simulink model "DoubleTankSim2023a"  (R2023a)
settings: Solver=ode5  StartTime=0.0  StopTime=250  RelTol=1e-3  EnableMultiTasking=on
values from neighbouring files (symbols this model uses):
  a1 = 0.145    [LeakSim.mat]    (also in disturbance.mat; main.m; mainLeak.m; out.mat)
  a2 = 0.145    [LeakSim.mat]    (also in disturbance.mat; main.m = 0.155; mainLeak.m; out.mat = 0.155)
  A_a = 33    [LeakSim.mat]    (also in disturbance.mat; main.m = 35; mainLeak.m; out.mat = 35)
  Ad = [0.997096423391  0  -0.448552524425; 0.00289935714461  0.997096423391  -0.000651834498432; 0  0  1]    [LeakSim.mat]    (also in disturbance.mat; out.mat = [0.998598500105  0; 0.00140036726045  0.998384495353]; out12.mat = [0.998598500105  0; 0.00140036726045  0.998384495353]; outLeak.mat = [0.998598500105  0; 0.00140036726045  0.998384495353])
  Bd = [0.0151295076986 2.19861321144e-05 0]    [LeakSim.mat]    (also in disturbance.mat; out.mat = [0.0107067759242 7.50574399214e-06]; out12.mat = [0.0107067759242 7.50574399214e-06]; outLeak.mat = [0.0107067759242 7.50574399214e-06])
  Cd = [0 1 0]    [LeakSim.mat]    (also in disturbance.mat; out.mat = [0 1]; out12.mat = [0 1]; outLeak.mat = [0 1])
  fh = [3 4 5 6 7 8 9 10 11 12 13 14 ... (13 elements, 1x13)]    [LeakSim.mat]    (also in disturbance.mat; main.m = [3 4 5 6 7 8 9 10 11 12 13 14 15]; mainLeak.m = [3 4 5 6 7 8 9 10 11 12 13 14 15]; out.mat)
  fq = [17.75 21.65 23.76 27.55 30.01 31.98 33.88 38.18 46.28 49.88]    [LeakSim.mat]    (also in disturbance.mat; main.m; mainLeak.m; out.mat)
  fu = [0.5 1 1.5 2 2.5 3 3.5 5 8 10]    [LeakSim.mat]    (also in disturbance.mat; main.m; mainLeak.m; out.mat)
  fv = [0.909 1.685 2.475 3.255 4.055 4.804 5.573 6.332 7.121 7.847 8.617 9.405 ... (13 elements, 1x13)]    [LeakSim.mat]    (also in disturbance.mat; main.m = [0.909 1.685 2.475 3.255 4.055 4.804 5.573 6.332 7.121 7.847; mainLeak.m = [0.909 1.685 2.475 3.255 4.055 4.804 5.573 6.332 7.121 7.847; out.mat)
  h0 = 3.2    [LeakSim.mat]    (also in disturbance.mat; main.m; mainLeak.m; out.mat)
  N = [1  0  0; 0  1  0; 0  0  1]    [LeakSim.mat]    (also in disturbance.mat; main.m = eye(2); mainLeak.m = eye(3); out.mat = [1  0; 0  1])
  P0 = [0  0  0; 0  0  0; 0  0  0]    [LeakSim.mat]    (also in disturbance.mat; main.m = zeros(2); mainLeak.m = zeros(3); out.mat = [0  0; 0  0])
  Q = [0.01  0  0; 0  0.01  0; 0  0  0.0001]    [LeakSim.mat]    (also in disturbance.mat; main.m = 0.1*eye(2); mainLeak.m = 0.01*eye(3,3); out.mat = [0.1  0; 0  0.1])
  R = 1e-06    [LeakSim.mat]    (also in disturbance.mat; main.m = Np*eye(2); mainLeak.m; out.mat = [0.0001  0; 0  0.0001])
  Ts = 0.1    [LeakSim.mat]    (also in disturbance.mat; main.m = 0.05; mainLeak.m; out.mat = 0.05)
  x0 = [-8 -8 0]    [LeakSim.mat]    (also in disturbance.mat; main.m = [0 0]'; mainLeak.m = [-8 -8 0]'; out.mat = [0 0])
undefined symbols (not defined in the file or in its folder): Continuous, Time
libraries: simulink x3, ctrlSharedLib x1
Description:
  | Double tank process simulation model
  | V1.0
  | 
  | Author: Wolfgang Birk, LTU
settings Model: MinMaxOverflowLogging=ForceOff  Creator=wolfgang  LastModifiedBy=vickay-0
settings SolverCC: AlgebraicLoopSolver=TrustRegion  AutoInsertRateTranBlk=on
settings DataIOCC: LimitDataPoints=on  SaveFormat=Array  SignalLoggingSaveFormat=ModelDataLogs  ReturnWorkspaceOutputs=off
settings OptimizationCC: ExpressionDepthLimit=2147483647  LifeSpan=inf
settings DebuggingCC: UnderspecifiedInitializationDetection=Classic  MergeDetectMultiDrivingBlocksExec=none  SolverPrmCheckMsg=warning  FcnCallInpInsideContextMsg=warning  UnconnectedInputMsg=warning  UnconnectedOutputMsg=warning  UnconnectedLineMsg=warning  StateNameClashWarn=warning  SFUnexpectedBacktrackingDiag=warning  SFNoUnconditionalDefaultTransitionDiag=warning  SFExecutionAtInitializationDiag=none  ArithmeticOperatorsInVariantConditions=warning
settings HardwareCC: ProdBitPerPointer=32  ProdBitPerSizeT=32  ProdBitPerPtrDiffT=32  ProdLargestAtomicFloat=None  ProdIntDivRoundTo=Undefined  ProdEndianess=Unspecified  ProdWordSize=32  ProdHWDeviceType=32-bit Generic
settings ModelReferenceCC: EnableRefExpFcnMdlSchedulingChecks=on  PropagateSignalLabelsOutOfModel=off
settings SFSimCC: SimUseLocalCustomCode=off  CustomCodeUndefinedFunction=UseInterfaceOnly
settings RTWCC: RTWUseLocalCustomCode=off
settings CodeAppCC: StateflowObjectComments=on
settings GRTTargetCC: TargetLangStandard=C89/C90 (ANSI)
settings ConfigComp: CovMetricSettings=dw  CovSaveCumulativeToWorkspaceVar=on  CovSaveSingleToWorkspaceVar=on  CovExternalEMLEnable=off

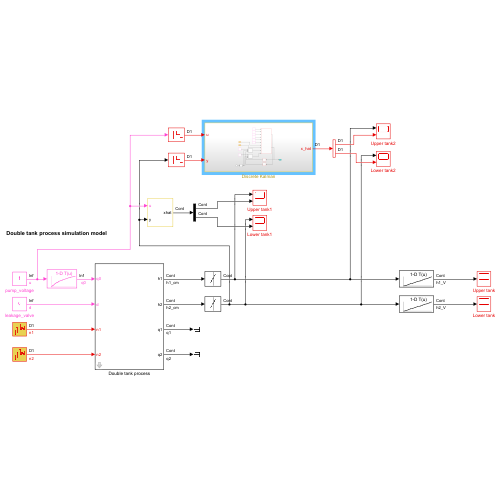
[thumbnail: Simulink's stored preview of the top-level diagram]
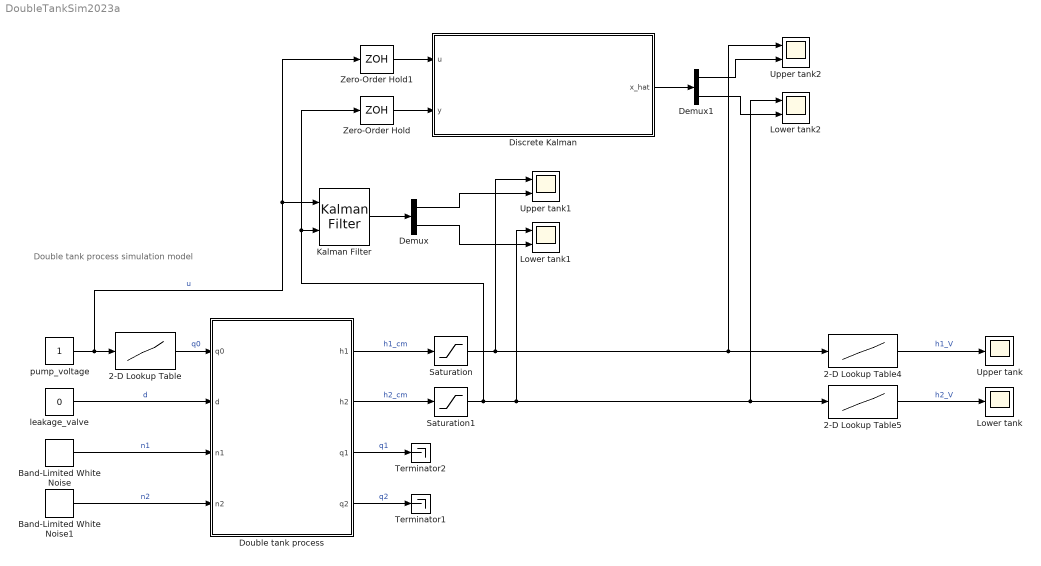
== system DoubleTankSim2023a ==
  note: Double tank process simulation model
  2-D Lookup Table : Lookup_n-D  NumberOfTableDimensions=1  BreakpointsForDimension1=x  BreakpointsForDimension2=[1:3]  Table=y  RndMeth=Simplest  mask{x=fu, y=fq}
      mask prompts: x "Values on x-axis"; y "Values on y-axis"
  2-D Lookup Table4 : Lookup_n-D  NumberOfTableDimensions=1  BreakpointsForDimension1=x  BreakpointsForDimension2=[1:3]  Table=y  RndMeth=Simplest  mask{x=fh, y=fv}
      mask prompts: x "Values on x-axis"; y "Values on y-axis"
  2-D Lookup Table5 : Lookup_n-D  NumberOfTableDimensions=1  BreakpointsForDimension1=x  BreakpointsForDimension2=[1:3]  Table=y  RndMeth=Simplest  mask{x=fh, y=fv}
      mask prompts: x "Values on x-axis"; y "Values on y-axis"
  Band-Limited White Noise : simulink/Sources/Band-Limited White Noise  Cov=Np  Ts=Ts  seed=[23341]
  Band-Limited White Noise1 : simulink/Sources/Band-Limited White Noise  Cov=Np  Ts=Ts  seed=[23341]
  Demux : Demux  Outputs=2
  Demux1 : Demux  Outputs=2
  Discrete Kalman : Subsystem
  Double tank process : Subsystem  mask{At=A_a, Ao=a1, hmax=15.5}
      mask prompts: At "Tank area (cm^2)"; Ao "Opening area (cm^2)"; hmax "Tank height (cm)"
      mask help: Double tank process parameters
  Kalman Filter : ctrlSharedLib/Kalman Filter  TimeDomain=Continuous-Time  UseCurrentEstimator=on  ModelSource=LTI State-Space Variable  ModelSourceVariable=sys  A=0.95  B=1  C=1  D=0  NumberOfStates=1  NumberOfInputs=1  NumberOfOutputs=1  InitialEstimateSource=Dialog  X0=0  P0=10  UseK=off  UseGH=off  NumberOfProcessNoiseInputs=1  G=1  TimeInvariantG=on  H=0  TimeInvariantH=on  Q=0  TimeInvariantQ=on  R=0.01  TimeInvariantR=on  N=0  TimeInvariantN=on  AddInputPort=on  AddEnablePort=off  OutputEstimatedY=off  OutputP=off  Ts=-1
  Lower tank : Scope
  Lower tank1 : Scope  NumInputPorts=2
  Lower tank2 : Scope  NumInputPorts=2
  Saturation : Saturate  UpperLimit=15.5  LowerLimit=3
  Saturation1 : Saturate  UpperLimit=15.5  LowerLimit=3
  Terminator1 : Terminator
  Terminator2 : Terminator
  Upper tank : Scope
  Upper tank1 : Scope  NumInputPorts=2
  Upper tank2 : Scope  NumInputPorts=2
  Zero-Order Hold : ZeroOrderHold  SampleTime=Ts
  Zero-Order Hold1 : ZeroOrderHold  SampleTime=Ts
  leakage_valve : Constant  Value=0
  pump_voltage : Constant
  wires:
  2-D Lookup Table4/1 -> Upper tank/1  "h1_V"
  leakage_valve/1 -> Double tank process/2(d)  "d"
  pump_voltage/1 -> Zero-Order Hold1/1, Kalman Filter/1, 2-D Lookup Table/1  "u"
  2-D Lookup Table/1 -> Double tank process/1(q0)  "q0"
  Double tank process/1(h1) -> Saturation/1  "h1_cm"
  Double tank process/2(h2) -> Saturation1/1  "h2_cm"
  Double tank process/4(q2) -> Terminator1/1  "q2"
  2-D Lookup Table5/1 -> Lower tank/1  "h2_V"
  Double tank process/3(q1) -> Terminator2/1  "q1"
  Band-Limited White Noise/1 -> Double tank process/3(n1)  "n1"
  Band-Limited White Noise1/1 -> Double tank process/4(n2)  "n2"
  Kalman Filter/1 -> Demux/1
  Demux/2 -> Lower tank1/2
  Demux/1 -> Upper tank1/2
  Saturation/1 -> Upper tank1/1, Upper tank2/1, 2-D Lookup Table4/1
  Saturation1/1 -> Zero-Order Hold/1, Kalman Filter/2, Lower tank1/1, Lower tank2/1, 2-D Lookup Table5/1
  Discrete Kalman/1(x_hat) -> Demux1/1
  Demux1/1 -> Upper tank2/2
  Demux1/2 -> Lower tank2/2
  Zero-Order Hold/1 -> Discrete Kalman/2(y)
  Zero-Order Hold1/1 -> Discrete Kalman/1(u)

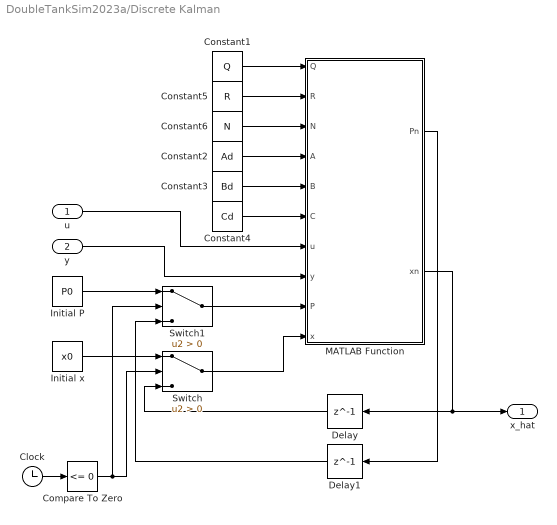
== system DoubleTankSim2023a/Discrete Kalman ==
  u : Inport  OutDataTypeStr=double  PortDimensions=1
  y : Inport  Port=2  OutDataTypeStr=double  PortDimensions=1
  Clock : Clock
  Compare To Zero : simulink/Logic and Bit Operations/Compare To Zero  relop=<=  OutDataTypeStr=boolean
  Constant1 : Constant  Value=Q  VectorParams1D=off
  Constant2 : Constant  Value=Ad  VectorParams1D=off
  Constant3 : Constant  Value=Bd  VectorParams1D=off
  Constant4 : Constant  Value=Cd  VectorParams1D=off
  Constant5 : Constant  Value=R  VectorParams1D=off
  Constant6 : Constant  Value=N  VectorParams1D=off
  Delay : Delay  DelayLength=1  InitialCondition=0  SampleTime=Ts
  Delay1 : Delay  DelayLength=1  InitialCondition=0  SampleTime=Ts
  Initial P : Constant  Value=P0
  Initial x : Constant  Value=x0
  MATLAB Function : MATLAB Function  TreatAsAtomicUnit=on  SystemSampleTime=Ts
  Switch : Switch  Criteria=u2 > Threshold  SaturateOnIntegerOverflow=off  InputSameDT=off
  Switch1 : Switch  Criteria=u2 > Threshold  SaturateOnIntegerOverflow=off  InputSameDT=off
  x_hat : Outport
  wires:
  Clock/1 -> Compare To Zero/1
  Initial x/1 -> Switch/1
  Compare To Zero/1 -> Switch/2, Switch1/2
  Switch1/1 -> MATLAB Function/9(P)
  Initial P/1 -> Switch1/1
  Delay1/1 -> Switch1/3
  Delay/1 -> Switch/3
  Switch/1 -> MATLAB Function/10(x)
  MATLAB Function/1(Pn) -> Delay1/1
  MATLAB Function/2(xn) -> x_hat/1, Delay/1
  y/1 -> MATLAB Function/8(y)
  u/1 -> MATLAB Function/7(u)
  Constant4/1 -> MATLAB Function/6(C)
  Constant3/1 -> MATLAB Function/5(B)
  Constant2/1 -> MATLAB Function/4(A)
  Constant6/1 -> MATLAB Function/3(N)
  Constant5/1 -> MATLAB Function/2(R)
  Constant1/1 -> MATLAB Function/1(Q)

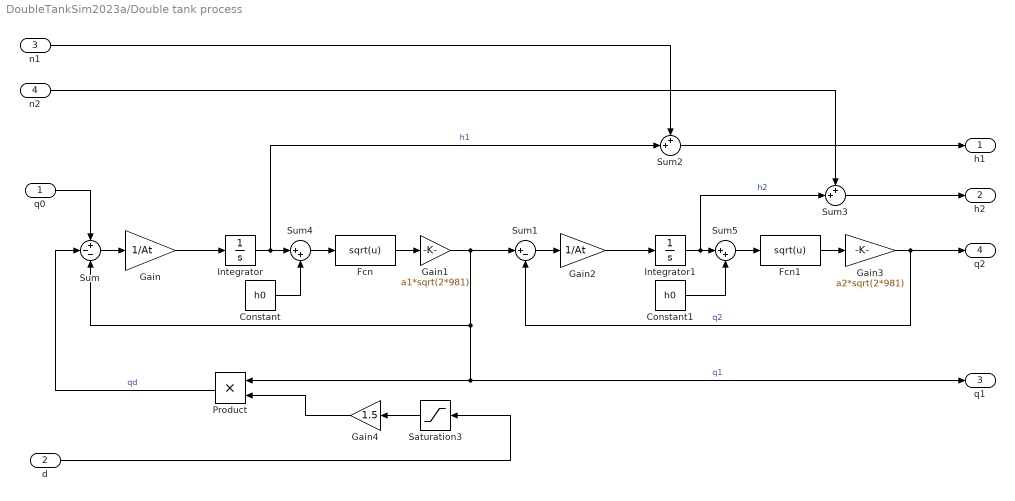
== system DoubleTankSim2023a/Double tank process ==
  q0 : Inport
  d : Inport  Port=2
  n1 : Inport  Port=3
  n2 : Inport  Port=4
  Constant : Constant  Value=h0
  Constant1 : Constant  Value=h0
  Fcn : Fcn  Expr=sqrt(u)
  Fcn1 : Fcn  Expr=sqrt(u)
  Gain : Gain  Gain=1/At
  Gain1 : Gain  Gain=a1*sqrt(2*981)
  Gain2 : Gain  Gain=1/At
  Gain3 : Gain  Gain=a2*sqrt(2*981)
  Gain4 : Gain  Gain=1.5
  Integrator : Integrator  LimitOutput=on  UpperSaturationLimit=hmax  LowerSaturationLimit=0
  Integrator1 : Integrator  LimitOutput=on  UpperSaturationLimit=hmax  LowerSaturationLimit=0
  Product : Product  RndMeth=Zero
  Saturation3 : Saturate  UpperLimit=1  LowerLimit=0
  Sum : Sum  Inputs=+--
  Sum1 : Sum  Inputs=|+-
  Sum2 : Sum  Inputs=++|
  Sum3 : Sum  Inputs=++|
  Sum4 : Sum  Inputs=|++
  Sum5 : Sum  Inputs=|++
  h1 : Outport  VectorParamsAs1DForOutWhenUnconnected=off
  h2 : Outport  Port=2  VectorParamsAs1DForOutWhenUnconnected=off
  q1 : Outport  Port=3  VectorParamsAs1DForOutWhenUnconnected=off
  q2 : Outport  Port=4  VectorParamsAs1DForOutWhenUnconnected=off
  wires:
  Sum/1 -> Gain/1
  Gain/1 -> Integrator/1
  Fcn/1 -> Gain1/1
  Gain1/1 -> Sum1/1, Product/1, q1/1, Sum/3  "q1"
  Sum1/1 -> Gain2/1
  Gain2/1 -> Integrator1/1
  Fcn1/1 -> Gain3/1
  Gain3/1 -> Sum1/2, q2/1  "q2"
  q0/1 -> Sum/1
  Integrator/1 -> Sum4/1, Sum2/2  "h1"
  Product/1 -> Sum/2  "qd"
  d/1 -> Saturation3/1
  Integrator1/1 -> Sum5/1, Sum3/2  "h2"
  Saturation3/1 -> Gain4/1
  Gain4/1 -> Product/2
  Sum2/1 -> h1/1
  n1/1 -> Sum2/1
  Sum3/1 -> h2/1
  n2/1 -> Sum3/1
  Sum4/1 -> Fcn/1
  Constant/1 -> Sum4/2
  Sum5/1 -> Fcn1/1
  Constant1/1 -> Sum5/2

== matlab function DoubleTankSim2023a/Discrete Kalman/MATLAB Function ==
  data: Q input; R input; N input; A input; B input; C input; u input; y input; P input; x input; Pn output; xn output
function [Pn,xn] = fcn(Q,R,N,A,B,C,u,y,P,x)

% Predict 
xn = A * x + B * u; 
Pn = A * P * A' + N*Q*N';

% Update 
K = (Pn * C') \ (C * Pn * C' + R); 
xn = xn + K * [0; (y - C * xn)]; Pn = Pn - K*C'*Pn;

end
